simulink model "cosimulation_simulink"  (R2025b)
settings: Solver=VariableStepAuto  StartTime=0.0  StopTime=3  RelTol=1e-3
libraries: fillib x1
settings Model: Creator=llillo  LastModifiedBy=llillo

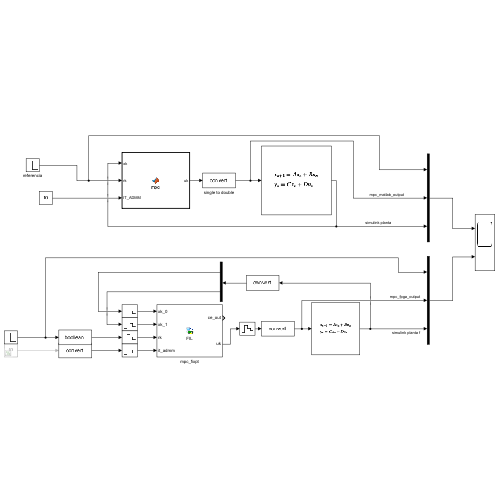
[thumbnail: Simulink's stored preview of the top-level diagram]
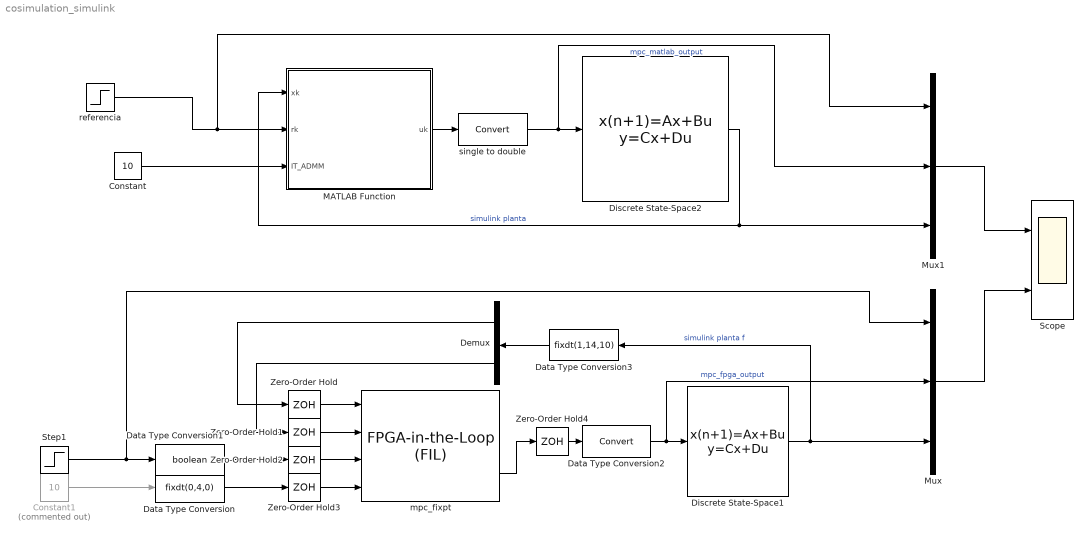
== system cosimulation_simulink ==
  Constant : Constant  Value=10  SampleTime=0.001
  Constant1 : Constant  Commented=on  Value=10  SampleTime=0.001
  Data Type Conversion : DataTypeConversion  OutDataTypeStr=fixdt(0,4,0)  SaturateOnIntegerOverflow=off  RndMeth=Floor
  Data Type Conversion1 : DataTypeConversion  OutDataTypeStr=boolean  SaturateOnIntegerOverflow=off  RndMeth=Floor  LockScale=on
  Data Type Conversion2 : DataTypeConversion  SaturateOnIntegerOverflow=off  RndMeth=Floor
  Data Type Conversion3 : DataTypeConversion  OutDataTypeStr=fixdt(1,14,10)  SaturateOnIntegerOverflow=off  RndMeth=Floor
  Demux : Demux  Outputs=2
  Discrete State-Space1 : DiscreteStateSpace  A=|  B=|  C=eye(2)  D=[0;0]  InitialCondition=[3; -1]  SampleTime=0.001
      A=|
      | [exp(-Ts/tau)                 0;
      |      tau*(1-exp(-Ts/tau))         1]
      B=|
      | [kappa*(1-exp(-Ts/tau));
      |      Ts*kappa + tau*kappa*(exp(-Ts/tau) - 1)]
  Discrete State-Space2 : DiscreteStateSpace  A=|  B=|  C=eye(2)  D=[0;0]  InitialCondition=[3; -1]  SampleTime=0.001
      A=|
      | [exp(-Ts/tau)                 0;
      |      tau*(1-exp(-Ts/tau))         1]
      B=|
      | [kappa*(1-exp(-Ts/tau));
      |      Ts*kappa + tau*kappa*(exp(-Ts/tau) - 1)]
  MATLAB Function : MATLAB Function  TreatAsAtomicUnit=on
  Mux : Mux  Inputs=3
  Mux1 : Mux  Inputs=3
  Scope : Scope  NumInputPorts=2
      settings: ActiveDisplayYMinimum=-4.0558876861567237  ActiveDisplayYMaximum=5.11380755510367
  Step1 : Step  Time=1.5  Before=1  After=0  SampleTime=0.001
  Zero-Order Hold{,1..4} (5 alike) : ZeroOrderHold  SampleTime=0.001
  mpc_fixpt : fillib/FPGA-in-the-Loop (FIL)  ForceInterfaceUpdate=0.81472
  referencia : Step  Time=1.5  Before=1  After=0  SampleTime=0.001
  single to double : DataTypeConversion  SaturateOnIntegerOverflow=off  RndMeth=Floor
  wires:
  MATLAB Function/1(uk) -> single to double/1
  Constant/1 -> MATLAB Function/3(IT_ADMM)
  Discrete State-Space2/1 -> Mux1/3, MATLAB Function/1(xk)  "simulink planta"
  referencia/1 -> Mux1/1, MATLAB Function/2(rk)
  Constant1/1 -> Data Type Conversion/1
  Discrete State-Space1/1 -> Data Type Conversion3/1, Mux/3  "simulink planta f"
  mpc_fixpt/2 -> Zero-Order Hold4/1
  Step1/1 -> Mux/1, Data Type Conversion1/1
  Data Type Conversion/1 -> Zero-Order Hold3/1
  Data Type Conversion1/1 -> Zero-Order Hold2/1
  Data Type Conversion3/1 -> Demux/1
  Demux/2 -> Zero-Order Hold1/1
  Demux/1 -> Zero-Order Hold/1
  Zero-Order Hold/1 -> mpc_fixpt/1
  Zero-Order Hold1/1 -> mpc_fixpt/2
  Zero-Order Hold2/1 -> mpc_fixpt/3
  Zero-Order Hold3/1 -> mpc_fixpt/4
  Zero-Order Hold4/1 -> Data Type Conversion2/1
  Mux1/1 -> Scope/1
  Mux/1 -> Scope/2
  Data Type Conversion2/1 -> Mux/2, Discrete State-Space1/1  "mpc_fpga_output"
  single to double/1 -> Mux1/2, Discrete State-Space2/1  "mpc_matlab_output"

== matlab function cosimulation_simulink/MATLAB Function ==
  data: xk input; uk output; rk input; IT_ADMM input
function uk = mpc(xk, rk, IT_ADMM)
%MPC Summary of this function goes here
%   Detailed explanation goes here

%format('longE')

N_HOR = 4;      % Tamaño del horizonte de predicción
%x0 = single([3.0; -1.0]);    % Velocidad y posición angular inicial

% Restricciones del sistema
umin = -3;
umax = 3;
xmin = [-5; -2];
xmax = [5; 2];

% Referencia deseada del sistema
%rk = zeros(1, length(k));
%rk(1, 1:1500) = rk(1, 1:1500) + 1;

%IT_ADMM = 10;

%% Formulación Densa

N_SYS = 2;
M_SYS = 1;
%P_SYS = 1;

%x0 = zeros(N_SYS, length(k), 'single');
%uk = zeros(M_SYS, length(k), 'single');
%xk(:, 1) = x0; % supongo que este es un warm start

%theta = zeros(N_QP, length(k), 'single');

%[D, E] = fx_dense_matrices(A, B, N_HOR);
%K = blkdiag(kron(eye(N_HOR - 1), Omega), OmegaN);
%L = kron(eye(N_HOR), Gamma); 
%Q = 2 * (L + E' * K * E);
%Q = (Q + Q') / 2;
%D = single(D);
%F = single(2 * D' * K * E); 
%G = [eye(N_QP); -eye(N_QP); E; -E];

%rho = single(fx_dhang_rho(Q, G));
%Q = single(Q);
%G = single(G);

D = [0.972466171 0;0.000986168976 1;0.945690453 0;0.00194518501 1;0.919651926 0;0.0028777956 1;0.894330382 0;0.00378472777 1];

F = [0.0214235317 0.0213781651 0.0213316325 0.0212839693;0.64161247 0.638990045 0.636372685 0.633760333];

T_inv = [-0.502326608 1000 0;0 0 1;25.5885372 714.431946 0];

%% Iteración MPC

%t_ADMM = zeros(N_QP, 1, 'single');
%z_ADMM = zeros(M_QP, 1, 'single');
%u_ADMM = zeros(M_QP, 1, 'single');

%for i = 1:length(k)%ESTE DEBERIA SER EL LLAMADO A MPC
    ref = [zeros(N_SYS,1,'single'); rk];
    inf = T_inv * ref;
    xinf = inf(1:N_SYS);
    uinf = inf(N_SYS+1 : N_SYS+M_SYS);
    q = ((xk - xinf)' * F)';
    c = repmat(umax - uinf, N_HOR, 1);
    d = repmat(umin - uinf, N_HOR, 1);
    e = repmat(xmax - xinf, N_HOR, 1);
    f = repmat(xmin - xinf, N_HOR, 1);
    g = [c; -d; e - D * xk; D * xk - f];
    %%
    t_ADMM = fx_qp_admm(q, g, IT_ADMM);
    uk = t_ADMM(1:M_SYS) + uinf;%ESTO VA GUARDANDO TODAS LAS SALIDAS
%end

end


%% QP SOLVER - ADMM
% ===============================================================================
% Alfonso Cortes Neira - Universidad Técnica Federico Santa María
% 16-02-2023
% Based on the work by Juan David Escárate
% ===============================================================================

function t  = fx_qp_admm(q, g, iters)          
% fx_qp_admm - Solución de un problema de optimización cuadrática con ADMM
N_SYS = 2;
M_SYS = 1;
N_HOR = 4;

N_QP = N_HOR * M_SYS;
M_QP = 2 * N_HOR * (N_SYS + M_SYS);

G = [1 0 0 0;0 1 0 0;0 0 1 0;0 0 0 1;-1 0 0 0;0 -1 0 0;0 0 -1 0;0 0 0 -1;0.0385394841 0 0 0;1.93594096e-05 0 0 0;0.0374783464 0.0385394841 0 0;5.73658581e-05 1.93594096e-05 0 0;0.0364464223 0.0374783464 0.0385394841 0;9.43258419e-05 5.73658581e-05 1.93594096e-05 0;0.0354429111 0.0364464223 0.0374783464 0.0385394841;0.000130268178 9.43258419e-05 5.73658581e-05 1.93594096e-05;-0.0385394841 0 0 0;-1.93594096e-05 0 0 0;-0.0374783464 -0.0385394841 0 0;-5.73658581e-05 -1.93594096e-05 0 0;-0.0364464223 -0.0374783464 -0.0385394841 0;-9.43258419e-05 -5.73658581e-05 -1.93594096e-05 0;-0.0354429111 -0.0364464223 -0.0374783464 -0.0385394841;-0.000130268178 -9.43258419e-05 -5.73658581e-05 -1.93594096e-05];

R_inv = [2.47927713 -0.0101672383 -0.00845972542 -0.00676105311;-0.0101672392 2.48085499 -0.00855126418 -0.00680351257;-0.00845972635 -0.00855126418 2.48251104 -0.00685224542;-0.00676105265 -0.00680351257 -0.00685224542 2.48425579];

P = [-0.100709476 0 0 0 0.100709476 0 0 0 -0.00388129125 -1.94967606e-06 -0.00377442455 -5.77728542e-06 -0.00367050013 -9.49950572e-06 -0.00356943696 -1.31192401e-05 0.00388129125 1.94967606e-06 0.00377442455 5.77728542e-06 0.00367050013 9.49950572e-06 0.00356943696 1.31192401e-05;0 -0.100709476 0 0 0 0.100709476 0 0 0 0 -0.00388129125 -1.94967606e-06 -0.00377442455 -5.77728542e-06 -0.00367050013 -9.49950572e-06 0 0 0.00388129125 1.94967606e-06 0.00377442455 5.77728542e-06 0.00367050013 9.49950572e-06;0 0 -0.100709476 0 0 0 0.100709476 0 0 0 0 0 -0.00388129125 -1.94967606e-06 -0.00377442455 -5.77728542e-06 0 0 0 0 0.00388129125 1.94967606e-06 0.00377442455 5.77728542e-06;0 0 0 -0.100709476 0 0 0 0.100709476 0 0 0 0 0 0 -0.00388129125 -1.94967606e-06 0 0 0 0 0 0 0.00388129125 1.94967606e-06];

% Min: 0.5*tk'*Q*tk + q'*tk
% Sujeto a: G*tk <= g

    % Verificar el número de argumentos de entrada
    %if nargin ~= 9
    %    error('ADMM_QP:incorrectInputs', 'Número incorrecto de entradas');
    %end

    % Inicialización de variables
    %tk = init_tk;
    %zk = init_zk;
    %uk = init_uk;
    persistent tk zk uk

    if isempty(tk)
        tk = zeros(N_QP, 1, 'single');
        zk = zeros(M_QP, 1, 'single');
        uk = zeros(M_QP, 1, 'single');
    end
    % Preparación de la matriz R y su inversa
    %R = Q + rho * (G' * G);
    %R_inv = R \ eye(size(R, 1));

    % Iteraciones de ADMM
    for k = 1:iters
        v_x = zk - g + uk;
        tk = R_inv * (P * v_x - q);  % Actualizar tk
        zk = max(0, -G * tk - uk + g);       % Actualizar zk
        uk = uk + (G * tk + zk - g);
    end
    t=tk;
end
